simulink model "elecmechsim"  (R2025a)
settings: Solver=FixedStepAuto  StartTime=0.0  StopTime=100  FixedStep=0.001  RelTol=1e-3
settings Model: Creator=Fishyman  LastModifiedBy=crice

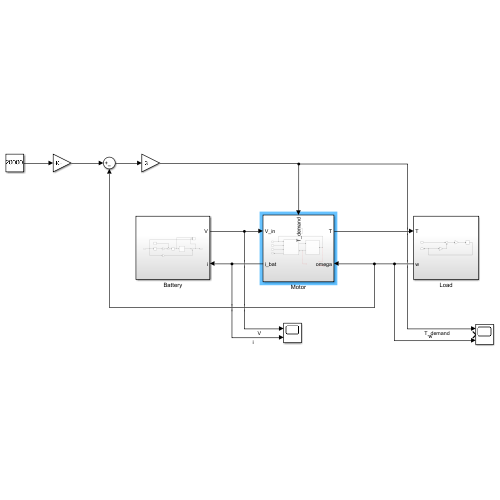
[thumbnail: Simulink's stored preview of the top-level diagram]
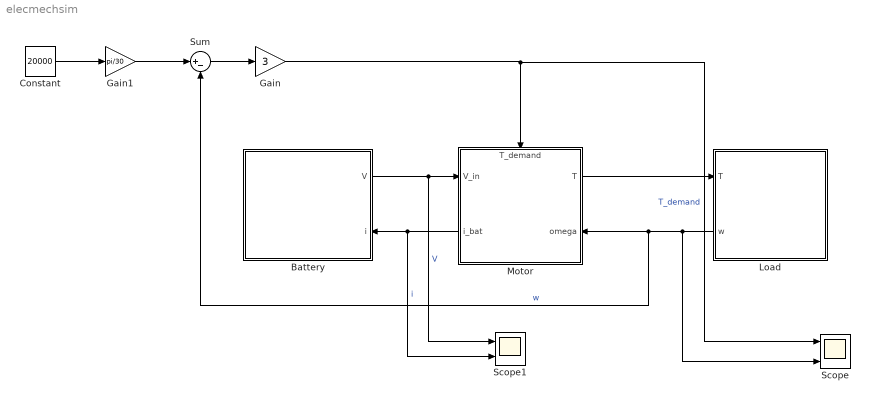
== system elecmechsim ==
  Battery : Subsystem
      settings: PortSchema="{\"entries\":[{\"content\":{\"sides\":[{\"content\":{},\"type\":\"ConnectorPlacement.EquallySpacedRectSide\",\"uuid\":\"90dd6bea-f724-4f0e-b388-4faa47577b06\"},{\"content\":{\"connectorIds\":[\"Out1\",\"In1\"],\"side\":\"RIGHT\"},\"type\":\"ConnectorPlacement.EquallySpacedRectSide\",\"uuid\":\"c3b6cbe3-b84f-419e-9715-7957d7ea1c1e\"},{\"content\":{\"side\":\"TOP\"},\"type\":\"ConnectorPlacement.EquallySpacedRectSide\",\"uuid\":\"193a9e4d-398d-403b-bf54-6d04e8a510a2\"}]},\"type\":\"ConnectorPlacement.EquallySpacedConnector\",\"uuid\":\"ee056e4f-358f-4828-90d3-6930ea0d5628\"}],\"packageUris\":[\"http://schema.mathworks.com/mf0/Connector/R2020b\"],\"version\":\"1.0\"}"
  Constant : Constant  Value=20000
  Gain : Gain  Gain=3
  Gain1 : Gain  Gain=pi/30
  Load : Subsystem
      settings: PortSchema="{\"entries\":[{\"content\":{\"sides\":[{\"content\":{\"connectorIds\":[\"In1\",\"Out1\"]},\"type\":\"ConnectorPlacement.EquallySpacedRectSide\",\"uuid\":\"90dd6bea-f724-4f0e-b388-4faa47577b06\"},{\"content\":{\"side\":\"RIGHT\"},\"type\":\"ConnectorPlacement.EquallySpacedRectSide\",\"uuid\":\"c3b6cbe3-b84f-419e-9715-7957d7ea1c1e\"},{\"content\":{\"side\":\"TOP\"},\"type\":\"ConnectorPlacement.EquallySpacedRectSide\",\"uuid\":\"193a9e4d-398d-403b-bf54-6d04e8a510a2\"}]},\"type\":\"ConnectorPlacement.EquallySpacedConnector\",\"uuid\":\"ee056e4f-358f-4828-90d3-6930ea0d5628\"}],\"packageUris\":[\"http://schema.mathworks.com/mf0/Connector/R2020b\"],\"version\":\"1.0\"}"
  Motor : Subsystem
      settings: PortSchema="{\"entries\":[{\"content\":{\"sides\":[{\"content\":{\"connectorIds\":[\"In1\",\"Out2\"]},\"type\":\"ConnectorPlacement.EquallySpacedRectSide\",\"uuid\":\"59bece3f-90cf-47e3-b7f7-45472b4ed29b\"},{\"content\":{\"connectorIds\":[\"Out1\",\"In3\"],\"side\":\"RIGHT\"},\"type\":\"ConnectorPlacement.EquallySpacedRectSide\",\"uuid\":\"a8762b20-55df-48c6-9a38-100f62965a72\"},{\"content\":{\"connectorIds\":[\"In2\"],\"side\":\"TOP\"},\"type\":\"ConnectorPlacement.EquallySpacedRectSide\",\"uuid\":\"f2b0052a-0f93-449a-a72f-4be1aa749add\"}]},\"type\":\"ConnectorPlacement.EquallySpacedConnector\",\"uuid\":\"3b29a972-b8e8-42da-9561-e1105daf668b\"}],\"packageUris\":[\"http://schema.mathworks.com/mf0/Connector/R2020b\"],\"version\":\"1.0\"}"
  Scope : Scope  NumInputPorts=3
      settings: ActiveDisplayYMinimum=5708.76635  ActiveDisplayYMaximum=6347.00964
  Scope1 : Scope  NumInputPorts=2
      settings: ActiveDisplayYMinimum=40.25471  ActiveDisplayYMaximum=42.74948
  Sum : Sum  Inputs=|+-
  wires:
  Battery/1(V) -> Scope1/1, Motor/1(V_in)  "V"
  Motor/2(i_bat) -> Scope1/2, Battery/1(i)  "i"
  Load/1(w) -> Scope/3, Sum/2, Motor/3(omega)  "w"
  Sum/1 -> Gain/1
  Constant/1 -> Gain1/1
  Gain/1 -> Scope/1, Motor/2(T_demand)  "T_demand"
  Gain1/1 -> Sum/1
  Motor/1(T) -> Load/1(T)

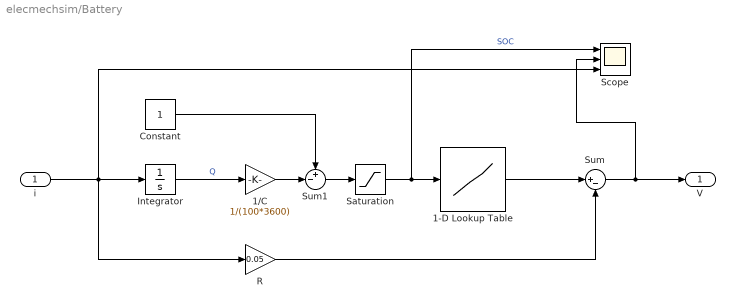
== system elecmechsim/Battery ==
  i : Inport
  1-D Lookup Table : Lookup_n-D  NumberOfTableDimensions=1  BreakpointsForDimension1=[0, 0.15, 0.2, 0.8, 0.95, 1]  Table=[22.5, 35, 37.5, 37.5, 40, 42.5]  InternalRulePriority=Speed  RndMeth=Simplest
  1/C : Gain  Gain=1/(100*3600)
  Constant : Constant
  Integrator : Integrator
  R : Gain  Gain=0.05
  Saturation : Saturate  UpperLimit=1  LowerLimit=0
  Scope : Scope  NumInputPorts=3
      settings: ActiveDisplayYMinimum=0.99078  ActiveDisplayYMaximum=1.00102  DataLoggingVariableName=ScopeData4
  Sum : Sum  Inputs=|+-
  Sum1 : Sum  Inputs=+-|
  V : Outport
  wires:
  Constant/1 -> Sum1/1
  i/1 -> R/1, Scope/3, Integrator/1
  1-D Lookup Table/1 -> Sum/1
  Integrator/1 -> 1/C/1  "Q"
  Saturation/1 -> Scope/1, 1-D Lookup Table/1  "SOC"
  Sum1/1 -> Saturation/1
  Sum/1 -> Scope/2, V/1
  1/C/1 -> Sum1/2
  R/1 -> Sum/2

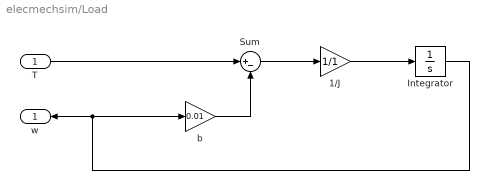
== system elecmechsim/Load ==
  T : Inport
  1/J : Gain  Gain=1/1
  Integrator : Integrator
  Sum : Sum  Inputs=|+-
  b : Gain  Gain=0.01
  w : Outport
  wires:
  1/J/1 -> Integrator/1
  Sum/1 -> 1/J/1
  Integrator/1 -> b/1, w/1
  T/1 -> Sum/1
  b/1 -> Sum/2

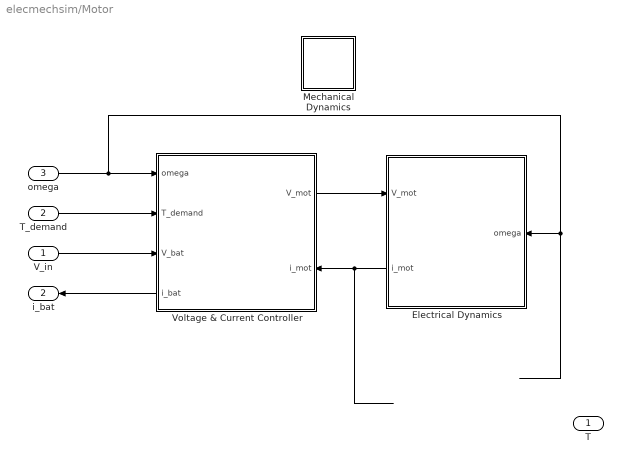
== system elecmechsim/Motor ==
  V_in : Inport
  T_demand : Inport  Port=2
  omega : Inport  Port=3
  Electrical Dynamics : Subsystem
      settings: PortSchema="{\"entries\":[{\"content\":{\"sides\":[{\"content\":{\"connectorIds\":[\"In1\",\"Out1\"]},\"type\":\"ConnectorPlacement.EquallySpacedRectSide\",\"uuid\":\"e446b3b9-b6cf-41bb-9ba1-a3aa4740c662\"},{\"content\":{\"connectorIds\":[\"In2\"],\"side\":\"RIGHT\"},\"type\":\"ConnectorPlacement.EquallySpacedRectSide\",\"uuid\":\"73556d2e-6dbd-43bd-8be5-c816eca01439\"},{\"content\":{\"side\":\"TOP\"},\"type\":\"ConnectorPlacement.EquallySpacedRectSide\",\"uuid\":\"80b3db30-baf9-488a-ad9e-05e46134b456\"},{\"content\":{\"side\":\"BOTTOM\"},\"type\":\"ConnectorPlacement.EquallySpacedRectSide\",\"uuid\":\"2369e07d-0029-49e3-9a6d-e102a23332b5\"}]},\"type\":\"ConnectorPlacement.EquallySpacedConnector\",\"uuid\":\"1c7cf443-8404-434d-b421-a5c7aaa92c5d\"}],\"packageUris\":[\"http://schema.mathworks.com/mf0/Connector/R2020b\"],\"version\":\"1.0\"}"
  Mechanical Dynamics : Subsystem
  Voltage & Current Controller : Subsystem
      settings: PortSchema="{\"entries\":[{\"content\":{\"sides\":[{\"content\":{\"connectorIds\":[\"In1\",\"In2\",\"In3\",\"Out2\"]},\"type\":\"ConnectorPlacement.EquallySpacedRectSide\",\"uuid\":\"7386bc59-c7cf-4e24-a03c-2c63c88805fb\"},{\"content\":{\"connectorIds\":[\"Out1\",\"In4\"],\"side\":\"RIGHT\"},\"type\":\"ConnectorPlacement.EquallySpacedRectSide\",\"uuid\":\"9d9f903b-7c00-446f-883d-5e6a0c4fe953\"},{\"content\":{\"side\":\"TOP\"},\"type\":\"ConnectorPlacement.EquallySpacedRectSide\",\"uuid\":\"243b84c1-c409-4364-aedd-e89918ead118\"}]},\"type\":\"ConnectorPlacement.EquallySpacedConnector\",\"uuid\":\"f42fac57-5517-4d2b-831b-44217276121d\"}],\"packageUris\":[\"http://schema.mathworks.com/mf0/Connector/R2020b\"],\"version\":\"1.0\"}"
  T : Outport
  i_bat : Outport  Port=2
  wires:
  V_in/1 -> Voltage & Current Controller/3(V_bat)
  T_demand/1 -> Voltage & Current Controller/2(T_demand)
  ? -> T/1
  Voltage & Current Controller/2(i_bat) -> i_bat/1
  Voltage & Current Controller/1(V_mot) -> Electrical Dynamics/1(V_mot)
  Electrical Dynamics/1(i_mot) -> Voltage & Current Controller/4(i_mot)
  omega/1 -> Electrical Dynamics/2(omega), Voltage & Current Controller/1(omega)

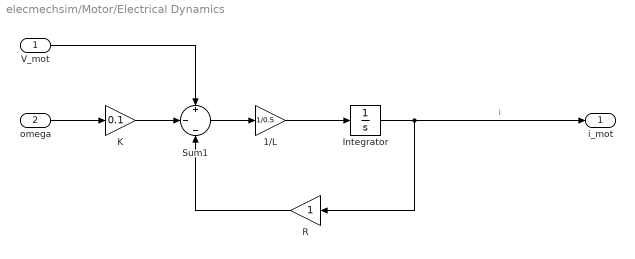
== system elecmechsim/Motor/Electrical Dynamics ==
  V_mot : Inport
  omega : Inport  Port=2
  1/L : Gain  Gain=1/0.5
  Integrator : Integrator
  K : Gain  Gain=0.1
  R : Gain
  Sum1 : Sum  Inputs=+|-|-
  i_mot : Outport
  wires:
  Integrator/1 -> R/1, i_mot/1  "i"
  Sum1/1 -> 1/L/1
  K/1 -> Sum1/2
  omega/1 -> K/1
  R/1 -> Sum1/3
  1/L/1 -> Integrator/1
  V_mot/1 -> Sum1/1

== system elecmechsim/Motor/Mechanical Dynamics ==

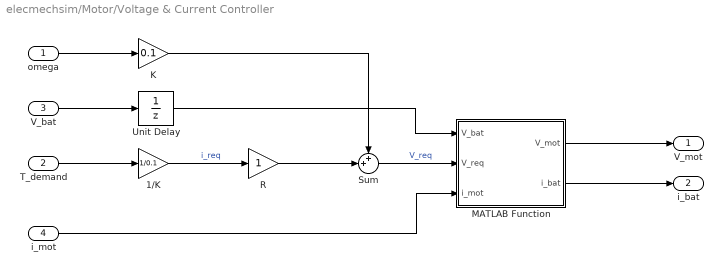
== system elecmechsim/Motor/Voltage & Current Controller ==
  omega : Inport
  T_demand : Inport  Port=2
  V_bat : Inport  Port=3
  i_mot : Inport  Port=4
  1/K : Gain  Gain=1/0.1
  K : Gain  Gain=0.1
  MATLAB Function : MATLAB Function  TreatAsAtomicUnit=on
  R : Gain
  Sum : Sum  Inputs=++|
  Unit Delay : UnitDelay  SampleTime=-1  HasFrameUpgradeWarning=on
  V_mot : Outport
  i_bat : Outport  Port=2
  wires:
  V_bat/1 -> Unit Delay/1
  R/1 -> Sum/2
  1/K/1 -> R/1  "i_req"
  K/1 -> Sum/1
  T_demand/1 -> 1/K/1
  omega/1 -> K/1
  Unit Delay/1 -> MATLAB Function/1(V_bat)
  Sum/1 -> MATLAB Function/2(V_req)  "V_req"
  i_mot/1 -> MATLAB Function/3(i_mot)
  MATLAB Function/1(V_mot) -> V_mot/1
  MATLAB Function/2(i_bat) -> i_bat/1

== matlab function elecmechsim/Motor/Voltage & Current Controller/MATLAB Function ==
  data: V_bat input; V_req input; V_mot output; i_mot input; i_bat output
function [V_mot, i_bat]= fcn(V_bat, V_req, i_mot)

V_mot = min(max(-V_bat, V_req), V_bat);
if V_bat == 0
    i_bat = 0;
else 
    i_bat = (V_mot * i_mot) / V_bat;
end
